simulink library "lib_sources"  (R2020b)
settings: Solver=VariableStepAuto  StartTime=0.0  StopTime=10.0  RelTol=1e-3
undefined symbols (not defined in the file): generator_polynomial
libraries: commseqgen3 x8, hdlsllib x1
settings Model: Creator=ckb13136  LastModifiedBy=ckb13136

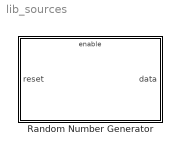
== system lib_sources ==
  Random Number Generator : Subsystem  mask{bits=8, gen_poly=generator_polynomial}
      mask prompts: bits "Data Bits:"; gen_poly "Generator Polynomial:"
      mask init:
      | random_gen = gcb;
      | 
      | set_param(random_gen, 'LinkStatus', 'none');
      | 
      | block_handles = Simulink.findBlocks(gcb);
      | block_names = getfullname(block_handles);
      | 
      | out_block = sprintf('%s/data', random_gen);
      | in_block = sprintf('%s/reset', random_gen);
      | enable_block = sprintf('%s/enable', random_gen);
      | 
      | keep_blocks = {out_block, in_block, enable_block};
      | 
      | for i = 1:length(block_names)
      |     if ~ismember(block_names{i}, keep_blocks)
      |         delete_block(block_names{i});
      |     end
      | end
      | delete_line(find_system(random_gen,'LookUnderMasks', 'all','FindAll','on','type','line'));
      | 
      | % Add all PN Sequence Generators 
      | for bit = 1:bits
      |     current_block = sprintf('%s/bit%d', random_gen, bit-1);
      |     add_block('commseqgen3/PN Sequence Generator', current_block);
      |     position = get_param(current_block, 'position');
      |     if bit == 1
      |         start_position = position;
      |     end
      |     new_position = position + ([0 60 0 60] * (bit-1));
      |     set_param(current_block, 'position', new_position);
      |     set_param(current_block, 'outDataType', 'boolean');
      |     set_param(current_block, 'reset', 'on');
      |     set_param(current_block, 'Ts', '-1');
      |     set_param(current_block, 'poly', gen_poly);
      |     
      |     val = dec2bin(randi(2^13 - 1), 13);
      |     str = '[';
      |     for i = 1:13
      |         str(end+1:end+2) = [' ' (val(i))];
      |     end
      |     str(end+1) = ']';
      |     set_param(current_block, 'ini_sta', str);
      | end
      | 
      | % Add the Bit Concat
      | concat_block = sprintf('%s/concat', random_gen);
      | add_block('hdlsllib/Logic and Bit Operations/Bit Concat', concat_block);
      | set_param(concat_block, 'numInputs', num2str(bits));
      | position = new_position + [150 0 150 0];
      | position(2) = start_position(2);
      | set_param(concat_block, 'position', position);
      | 
      | % Add Input and Outputs
      | out_position = get_param(out_block, 'position');
      | height = out_position(4) - out_position(2);
      | width = out_position(3) - out_position(1);
      | middle_h = (position(4) - position(2))/2 + position(2);
      | out_position = [position(1) + 150, middle_h - height/2, position(1) + 150 + width, middle_h + height/2];
      | set_param(out_block, 'position', out_position);
      | 
      | in_position = [position(1) - 300, middle_h - height/2, position(1) - 300 + width, middle_h + height/2];
      | set_param(in_block, 'position', in_position);
      | 
      | enable_position = get_param(enable_block, 'position');
      | set_param(enable_block, 'position', enable_position - [0 100 0 100]);
      | 
      | % Connect Ports
      | for bit = 1:bits
      |     add_line(random_gen,'reset/1', sprintf('bit%d/1', bit-1));
      |     add_line(random_gen,sprintf('bit%d/1', bit-1), sprintf('concat/%d', bit));
      | end
      | add_line(random_gen,'concat/1','data/1');
      mask DialogControl DescGroupVar Prompt: N-Bit Random Number Generator
      mask DialogControl DescTextVar Prompt: This block will create a n-bit random number generator. Provide a polynomial and the number of bits. Information on polynomials for maximal LFSRs can be found:  https://en.wikipedia.org/wiki/Linear-feedback_shift_register For example: ''z^13 + z^12 + z^11 + z^8 + 1''

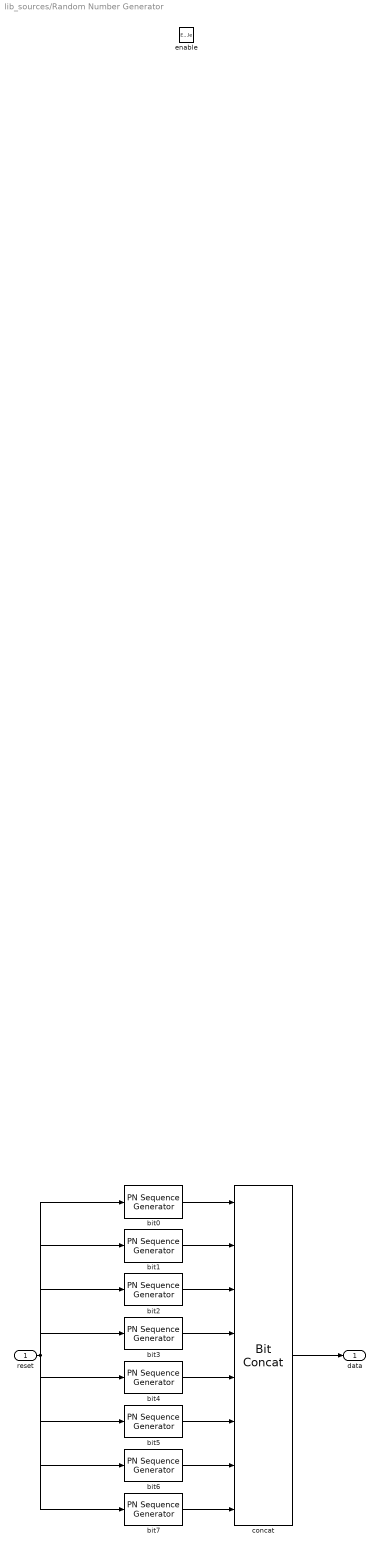
== system lib_sources/Random Number Generator ==
  reset : Inport
  enable : EnablePort
  bit0 : commseqgen3/PN Sequence Generator  poly='z^13 + z^12 + z^11 + z^8 + 1'  ini_sta=[ 0 0 1 0 0 1 0 0 0 1 0 1 1]  outBitMaskSource=Dialog parameter  shift=0  outVarSiz=off  maxOutSizeMode=Dialog parameter  maxOutSize=[10 1]  Ts=-1  sampPerFrame=1  reset=on  bitPackedOutputs=off  outDataType=boolean  numPackedBits=8  bitPackDataSigned=off  bitPackedOutDType=double
  bit1 : commseqgen3/PN Sequence Generator  poly='z^13 + z^12 + z^11 + z^8 + 1'  ini_sta=[ 0 1 1 0 1 0 1 1 1 1 1 1 1]  outBitMaskSource=Dialog parameter  shift=0  outVarSiz=off  maxOutSizeMode=Dialog parameter  maxOutSize=[10 1]  Ts=-1  sampPerFrame=1  reset=on  bitPackedOutputs=off  outDataType=boolean  numPackedBits=8  bitPackDataSigned=off  bitPackedOutDType=double
  bit2 : commseqgen3/PN Sequence Generator  poly='z^13 + z^12 + z^11 + z^8 + 1'  ini_sta=[ 1 1 1 0 1 0 1 0 0 1 1 0 1]  outBitMaskSource=Dialog parameter  shift=0  outVarSiz=off  maxOutSizeMode=Dialog parameter  maxOutSize=[10 1]  Ts=-1  sampPerFrame=1  reset=on  bitPackedOutputs=off  outDataType=boolean  numPackedBits=8  bitPackDataSigned=off  bitPackedOutDType=double
  bit3 : commseqgen3/PN Sequence Generator  poly='z^13 + z^12 + z^11 + z^8 + 1'  ini_sta=[ 1 1 0 0 1 0 1 0 1 1 0 0 1]  outBitMaskSource=Dialog parameter  shift=0  outVarSiz=off  maxOutSizeMode=Dialog parameter  maxOutSize=[10 1]  Ts=-1  sampPerFrame=1  reset=on  bitPackedOutputs=off  outDataType=boolean  numPackedBits=8  bitPackDataSigned=off  bitPackedOutDType=double
  bit4 : commseqgen3/PN Sequence Generator  poly='z^13 + z^12 + z^11 + z^8 + 1'  ini_sta=[ 1 1 1 1 0 1 0 1 1 0 1 0 0]  outBitMaskSource=Dialog parameter  shift=0  outVarSiz=off  maxOutSizeMode=Dialog parameter  maxOutSize=[10 1]  Ts=-1  sampPerFrame=1  reset=on  bitPackedOutputs=off  outDataType=boolean  numPackedBits=8  bitPackDataSigned=off  bitPackedOutDType=double
  bit5 : commseqgen3/PN Sequence Generator  poly='z^13 + z^12 + z^11 + z^8 + 1'  ini_sta=[ 1 0 1 0 0 1 1 1 1 1 1 0 0]  outBitMaskSource=Dialog parameter  shift=0  outVarSiz=off  maxOutSizeMode=Dialog parameter  maxOutSize=[10 1]  Ts=-1  sampPerFrame=1  reset=on  bitPackedOutputs=off  outDataType=boolean  numPackedBits=8  bitPackDataSigned=off  bitPackedOutDType=double
  bit6 : commseqgen3/PN Sequence Generator  poly='z^13 + z^12 + z^11 + z^8 + 1'  ini_sta=[ 0 0 0 0 1 0 0 1 0 0 1 0 1]  outBitMaskSource=Dialog parameter  shift=0  outVarSiz=off  maxOutSizeMode=Dialog parameter  maxOutSize=[10 1]  Ts=-1  sampPerFrame=1  reset=on  bitPackedOutputs=off  outDataType=boolean  numPackedBits=8  bitPackDataSigned=off  bitPackedOutDType=double
  bit7 : commseqgen3/PN Sequence Generator  poly='z^13 + z^12 + z^11 + z^8 + 1'  ini_sta=[ 1 1 0 1 1 0 0 1 0 1 1 0 0]  outBitMaskSource=Dialog parameter  shift=0  outVarSiz=off  maxOutSizeMode=Dialog parameter  maxOutSize=[10 1]  Ts=-1  sampPerFrame=1  reset=on  bitPackedOutputs=off  outDataType=boolean  numPackedBits=8  bitPackDataSigned=off  bitPackedOutDType=double
  concat : hdlsllib/Logic and Bit Operations/Bit Concat  numInputs=8
  data : Outport
  wires:
  reset/1 -> bit0/1, bit1/1, bit2/1, bit3/1, bit4/1, bit5/1, bit6/1, bit7/1
  bit0/1 -> concat/1
  bit1/1 -> concat/2
  bit2/1 -> concat/3
  bit3/1 -> concat/4
  bit4/1 -> concat/5
  bit5/1 -> concat/6
  bit6/1 -> concat/7
  bit7/1 -> concat/8
  concat/1 -> data/1
